simulink model "sim"  (R2017b)
settings: Solver=VariableStepAuto  StartTime=0.0  StopTime=Tsym  RelTol=1e-3
values from neighbouring files (symbols this model uses):
  Tn = 12    [pr_1.m]
  Ts = 2    [pr_1.m]
settings Model: Creator=BottomQuark  LastModifiedBy=piopi
settings DataIOCC: ReturnWorkspaceOutputs=on
settings SFSimCC: SimUseLocalCustomCode=on
settings RTWCC: RTWUseLocalCustomCode=on

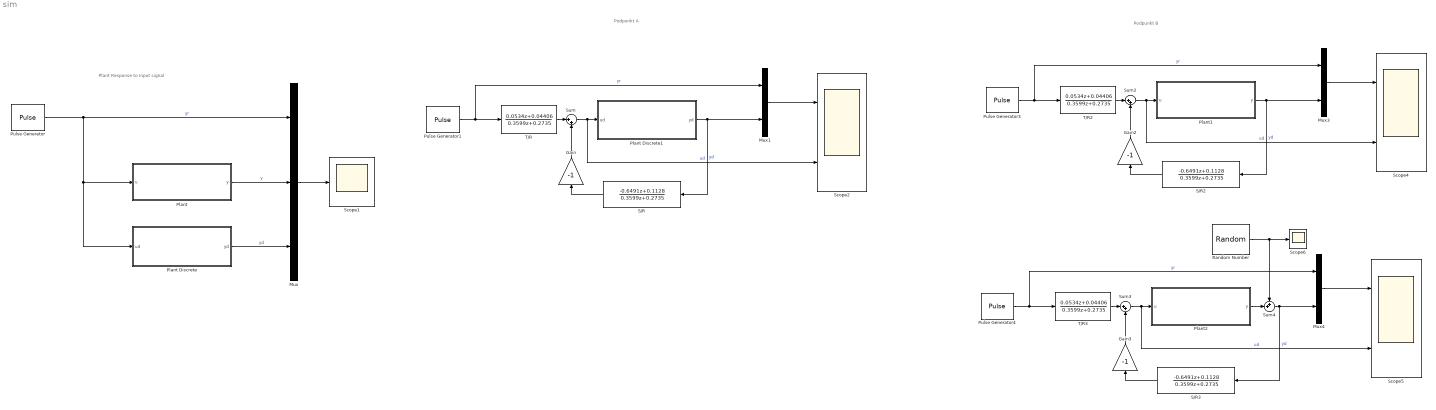
== system sim ==
  note: Plant Response to Input signal
  note: Podpunkt A
  note: Podpunkt B
  Gain : Gain  Gain=-1
  Gain2 : Gain  Gain=-1
  Gain3 : Gain  Gain=-1
  Mux : Mux  Inputs=3
  Mux1 : Mux  Inputs=2
  Mux3 : Mux  Inputs=2
  Mux4 : Mux  Inputs=2
  Plant : Subsystem
  Plant Discrete : Subsystem
  Plant Discrete1 : Subsystem
  Plant1 : Subsystem
  Plant2 : Subsystem
  Pulse Generator{,1,3..4} (4 alike) : DiscretePulseGenerator  PulseType=Time based  Period=20*Tn  PulseWidth=50
  Random Number : RandomNumber  Variance=0.003  SampleTime=0.1
  S/R : DiscreteTransferFcn  Numerator=[-0.6491, 0.1128]  Denominator=[0.3599, 0.2735]  SampleTime=Ts
  S/R2 : DiscreteTransferFcn  Numerator=[-0.6491, 0.1128]  Denominator=[0.3599, 0.2735]  SampleTime=Ts
  S/R3 : DiscreteTransferFcn  Numerator=[-0.6491, 0.1128]  Denominator=[0.3599, 0.2735]  SampleTime=Ts
  Scope1 : Scope
  Scope2 : Scope  NumInputPorts=2
  Scope4 : Scope  NumInputPorts=2
  Scope5 : Scope  NumInputPorts=2
  Scope6 : Scope
  Sum : Sum  Inputs=|++
  Sum2 : Sum  Inputs=|++
  Sum3 : Sum  Inputs=|++
  Sum4 : Sum  Inputs=++|
  T/R : DiscreteTransferFcn  Numerator=[0.0534, 0.04406]  Denominator=[0.3599, 0.2735]  SampleTime=Ts
  T/R2 : DiscreteTransferFcn  Numerator=[0.0534, 0.04406]  Denominator=[0.3599, 0.2735]  SampleTime=Ts
  T/R3 : DiscreteTransferFcn  Numerator=[0.0534, 0.04406]  Denominator=[0.3599, 0.2735]  SampleTime=Ts
  wires:
  Mux/1 -> Scope1/1
  Pulse Generator/1 -> Plant/1(u), Plant Discrete/1(ud), Mux/1  "yr"
  Plant/1(y) -> Mux/2  "y"
  Plant Discrete/1(yd) -> Mux/3  "yd"
  Pulse Generator1/1 -> Mux1/1, T/R/1  "yr"
  T/R/1 -> Sum/1
  Sum/1 -> Scope2/2, Plant Discrete1/1(ud)  "ud"
  Gain/1 -> Sum/2
  S/R/1 -> Gain/1
  Plant Discrete1/1(yd) -> Mux1/2, S/R/1  "yd"
  Mux1/1 -> Scope2/1
  Sum2/1 -> Plant1/1(u), Scope4/2  "ud"
  Mux3/1 -> Scope4/1
  T/R2/1 -> Sum2/1
  Plant1/1(y) -> Mux3/2, S/R2/1  "yd"
  Gain2/1 -> Sum2/2
  Pulse Generator3/1 -> Mux3/1, T/R2/1  "yr"
  S/R2/1 -> Gain2/1
  Plant2/1(y) -> Sum4/2
  Mux4/1 -> Scope5/1
  Pulse Generator4/1 -> Mux4/1, T/R3/1  "yr"
  T/R3/1 -> Sum3/1
  S/R3/1 -> Gain3/1
  Sum3/1 -> Plant2/1(u), Scope5/2  "ud"
  Gain3/1 -> Sum3/2
  Sum4/1 -> S/R3/1, Mux4/2  "yd"
  Random Number/1 -> Scope6/1, Sum4/1

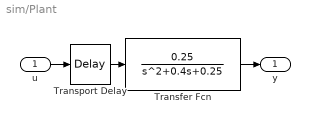
== system sim/Plant ==
  u : Inport
  Transfer Fcn : TransferFcn  Numerator=[0.25]  Denominator=[1 0.4 0.25]
  Transport Delay : TransportDelay  DelayTime=2
  y : Outport  VectorParamsAs1DForOutWhenUnconnected=on
  wires:
  Transport Delay/1 -> Transfer Fcn/1
  Transfer Fcn/1 -> y/1
  u/1 -> Transport Delay/1

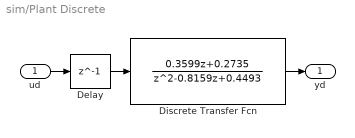
== system sim/Plant Discrete ==
  ud : Inport
  Delay : Delay  DelayLength=1  SampleTime=Ts
  Discrete Transfer Fcn : DiscreteTransferFcn  Numerator=[0.3599 0.2735]  Denominator=[1 -0.8159 0.4493]  SampleTime=Ts
  yd : Outport  VectorParamsAs1DForOutWhenUnconnected=on
  wires:
  Delay/1 -> Discrete Transfer Fcn/1
  ud/1 -> Delay/1
  Discrete Transfer Fcn/1 -> yd/1

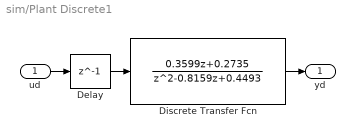
== system sim/Plant Discrete1 ==
  ud : Inport
  Delay : Delay  DelayLength=1  SampleTime=Ts
  Discrete Transfer Fcn : DiscreteTransferFcn  Numerator=[0.3599 0.2735]  Denominator=[1 -0.8159 0.4493]  SampleTime=Ts
  yd : Outport  VectorParamsAs1DForOutWhenUnconnected=on
  wires:
  Delay/1 -> Discrete Transfer Fcn/1
  ud/1 -> Delay/1
  Discrete Transfer Fcn/1 -> yd/1

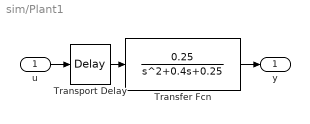
== system sim/Plant1 ==
  u : Inport
  Transfer Fcn : TransferFcn  Numerator=[0.25]  Denominator=[1 0.4 0.25]
  Transport Delay : TransportDelay  DelayTime=2
  y : Outport  VectorParamsAs1DForOutWhenUnconnected=on
  wires:
  Transport Delay/1 -> Transfer Fcn/1
  Transfer Fcn/1 -> y/1
  u/1 -> Transport Delay/1

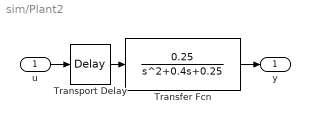
== system sim/Plant2 ==
  u : Inport
  Transfer Fcn : TransferFcn  Numerator=[0.25]  Denominator=[1 0.4 0.25]
  Transport Delay : TransportDelay  DelayTime=2
  y : Outport  VectorParamsAs1DForOutWhenUnconnected=on
  wires:
  Transport Delay/1 -> Transfer Fcn/1
  Transfer Fcn/1 -> y/1
  u/1 -> Transport Delay/1
